simulink model "pt8612_analog_pll"  (Simulink 5.0)
settings: Solver=ode45  StartTime=0.0  StopTime=35  MaxStep=1e-4  RelTol=1e-10  AbsTol=1e-13
values from neighbouring files (symbols this model uses):
  A = [[-1/Cp*(1/Rs+1/Rp) 1/Cp/Rs] ... (first row only)    [pt8612_analog_pll_init.m]    (also in pt8612_analog_pll_init_2.m = [[-1/C1/Ri     1/C1/Ri          0   ])
  B = [1/Cp 0].'    [pt8612_analog_pll_init.m]    (also in pt8612_analog_pll_init_2.m = [1/C1 0 0].')
  C = 680e-9    (= 6.8e-07)    [DPLL_init_2.m]    (also in pt8612_analog_pll_init.m = [1 0]; pt8612_analog_pll_init_2.m = [0 1 0]; pt8612_dpll_fpga_init.m; pt8612_dpll_fpga_init_2.m)
  fvcxo = 148.5e6/1.001    (= 148351648.352)    [DPLL_init_2.m]    (also in pt8612_analog_pll_init.m; pt8612_analog_pll_init_2.m; pt8612_dpll_fpga_init.m; pt8612_dpll_fpga_init_2.m = 148500000)
  Kvcxo = 90e-6    (= 9e-05)    [DPLL_init_2.m]    (also in pt8612_analog_pll_init.m; pt8612_analog_pll_init_2.m; pt8612_dpll_fpga_init.m; pt8612_dpll_fpga_init_2.m)
  Ndec1 = 91    [DPLL_init_2.m]    (also in pt8612_analog_pll_init.m; pt8612_analog_pll_init_2.m; pt8612_dpll_fpga_init.m = 364)
  Ndec2 = 500    [DPLL_init_2.m]    (also in pt8612_analog_pll_init.m; pt8612_analog_pll_init_2.m; pt8612_dpll_fpga_init.m = 2000)
  Ri = 100e3    (= 100000)    [pt8612_analog_pll_init.m]    (also in pt8612_analog_pll_init_2.m)
  Vcc = 3.3    [DPLL_init_2.m]    (also in pt8612_analog_pll_init.m; pt8612_analog_pll_init_2.m; pt8612_dpll_fpga_init.m = 2.5; pt8612_dpll_fpga_init_2.m = 2.5)
  Vvcxo0 = 1.25    [DPLL_init_2.m]    (also in pt8612_analog_pll_init.m; pt8612_analog_pll_init_2.m; pt8612_dpll_fpga_init.m; pt8612_dpll_fpga_init_2.m)
  Vvcxomax = 2.5    [DPLL_init_2.m]    (also in pt8612_analog_pll_init.m; pt8612_analog_pll_init_2.m; pt8612_dpll_fpga_init.m; pt8612_dpll_fpga_init_2.m)
  Vvcxomin = 0    [DPLL_init_2.m]    (also in pt8612_analog_pll_init.m; pt8612_analog_pll_init_2.m; pt8612_dpll_fpga_init.m; pt8612_dpll_fpga_init_2.m)
libraries: simulink x2
settings Model: LastModifiedBy=thh

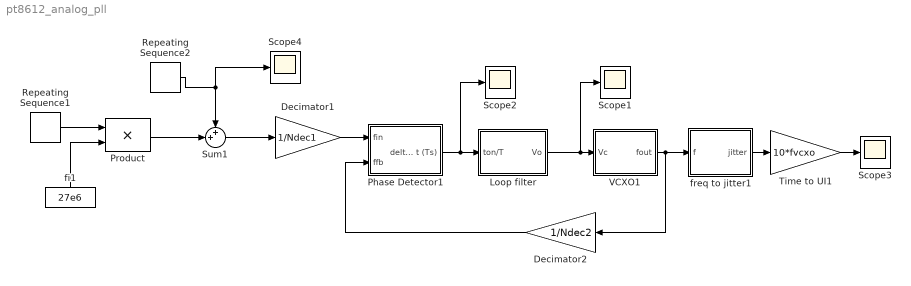
== system pt8612_analog_pll ==
  Decimator1 : Gain  Gain=1/Ndec1  SaturateOnIntegerOverflow=on
  Decimator2 : Gain  Orientation=left  Gain=1/Ndec2  SaturateOnIntegerOverflow=on
  Loop filter : Subsystem
  Phase Detector1 : Subsystem
  Product : Product  SaturateOnIntegerOverflow=on
  Repeating Sequence1 : simulink/Sources/Repeating Sequence  rep_seq_t=[0 10 10 20]  rep_seq_y=1+([0 0 30 30]*1e-6)*0
  Repeating Sequence2 : simulink/Sources/Repeating Sequence  rep_seq_t=[0 8-1e-3 8-1e-3 8 8 16-1e-3 16-1e-3 16]  rep_seq_y=[0 0 1 1 0 0 -1 -1]*30*1e3
  Scope{1..4} (4 alike) : Scope
      Scope1 settings: TimeRange=13.94281180037974  YMin=4.87505  YMax=5.12826
      Scope2 settings: TimeRange=13.94281180037974  YMin=0.05  YMax=0.75
      Scope3 settings: TimeRange=13.94281180037974  YMin=15  YMax=27  SaveName=ScopeData4
      Scope4 settings: TimeRange=13.94281180037974  YMin=-1  YMax=1  SaveName=ScopeData2
  Sum1 : Sum  Inputs=++|  SaturateOnIntegerOverflow=on
  Time to UI1 : Gain  Gain=10*fvcxo  SaturateOnIntegerOverflow=on
  VCXO1 : Subsystem
  fi1 : Constant  Orientation=up  Value=27e6
  freq to jitter1 : Subsystem
  wires:
  freq to jitter1/1(jitter) -> Time to UI1/1
  Time to UI1/1 -> Scope3/1
  Loop filter/1(Vo) -> VCXO1/1(Vc), Scope1/1
  VCXO1/1(fout) -> freq to jitter1/1(f), Decimator2/1
  Decimator2/1 -> Phase Detector1/2(ffb)
  fi1/1 -> Product/2
  Repeating Sequence1/1 -> Product/1
  Phase Detector1/1(delta t (Ts)) -> Loop filter/1(ton/T), Scope2/1
  Decimator1/1 -> Phase Detector1/1(fin)
  Repeating Sequence2/1 -> Sum1/1, Scope4/1
  Product/1 -> Sum1/2
  Sum1/1 -> Decimator1/1

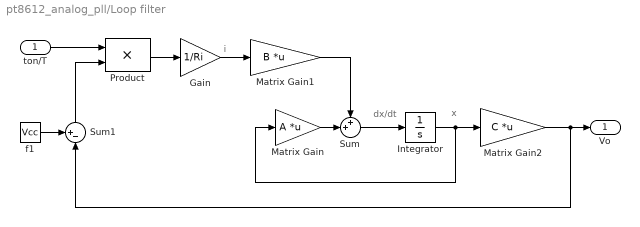
== system pt8612_analog_pll/Loop filter ==
  note: x
  note: dx/dt
  note: i
  ton/T : Inport
  Gain : Gain  Gain=1/Ri  SaturateOnIntegerOverflow=on
  Integrator : Integrator  InitialCondition=[1.25 1.25].'
  Matrix Gain : Gain  Gain=A  Multiplication=Matrix(K*u) (u vector)  SaturateOnIntegerOverflow=on
  Matrix Gain1 : Gain  Gain=B  Multiplication=Matrix(K*u)  SaturateOnIntegerOverflow=on
  Matrix Gain2 : Gain  Gain=C  Multiplication=Matrix(K*u) (u vector)  SaturateOnIntegerOverflow=on
  Product : Product  SaturateOnIntegerOverflow=on
  Sum : Sum  Inputs=++|  SaturateOnIntegerOverflow=on
  Sum1 : Sum  Orientation=up  Inputs=+-|  SaturateOnIntegerOverflow=on
  f1 : Constant  Value=Vcc
  Vo : Outport
  wires:
  Integrator/1 -> Matrix Gain2/1, Matrix Gain/1
  Sum/1 -> Integrator/1
  Matrix Gain/1 -> Sum/2
  Matrix Gain1/1 -> Sum/1
  Gain/1 -> Matrix Gain1/1
  Product/1 -> Gain/1
  Sum1/1 -> Product/2
  Matrix Gain2/1 -> Sum1/2, Vo/1
  f1/1 -> Sum1/1
  ton/T/1 -> Product/1

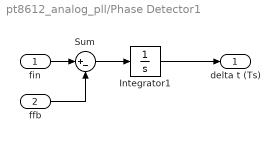
== system pt8612_analog_pll/Phase Detector1 ==
  fin : Inport
  ffb : Inport  Port=2
  Integrator1 : Integrator  InitialCondition=0.062
  Sum : Sum  Inputs=|+-  SaturateOnIntegerOverflow=on
  delta t (Ts) : Outport
  wires:
  Integrator1/1 -> delta t (Ts)/1
  ffb/1 -> Sum/2
  fin/1 -> Sum/1
  Sum/1 -> Integrator1/1

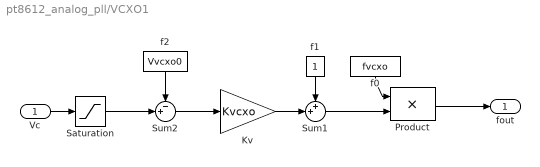
== system pt8612_analog_pll/VCXO1 ==
  Vc : Inport
  Kv : Gain  Gain=Kvcxo  SaturateOnIntegerOverflow=on
  Product : Product  SaturateOnIntegerOverflow=on
  Saturation : Saturate  UpperLimit=Vvcxomax  LowerLimit=Vvcxomin
  Sum1 : Sum  Inputs=++|  SaturateOnIntegerOverflow=on
  Sum2 : Sum  Inputs=-+|  SaturateOnIntegerOverflow=on
  f0 : Constant  Orientation=down  Value=fvcxo
  f1 : Constant  Orientation=down
  f2 : Constant  Orientation=down  Value=Vvcxo0
  fout : Outport
  wires:
  f2/1 -> Sum2/1
  Vc/1 -> Saturation/1
  Sum2/1 -> Kv/1
  Product/1 -> fout/1
  Kv/1 -> Sum1/2
  Sum1/1 -> Product/2
  f1/1 -> Sum1/1
  f0/1 -> Product/1
  Saturation/1 -> Sum2/2

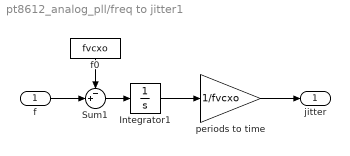
== system pt8612_analog_pll/freq to jitter1 ==
  f : Inport
  Integrator1 : Integrator
  Sum1 : Sum  Inputs=-+|  SaturateOnIntegerOverflow=on
  f0 : Constant  Orientation=down  Value=fvcxo
  periods to time : Gain  Gain=1/fvcxo  SaturateOnIntegerOverflow=on
  jitter : Outport
  wires:
  periods to time/1 -> jitter/1
  f/1 -> Sum1/2
  f0/1 -> Sum1/1
  Sum1/1 -> Integrator1/1
  Integrator1/1 -> periods to time/1
